simulink model "sim_task_2"  (R2024a)
settings: Solver=FixedStepAuto  StartTime=0.0  StopTime=10.0  FixedStep=1e-3  RelTol=1e-3
settings Model: Creator=alexe  LastModifiedBy=alexe

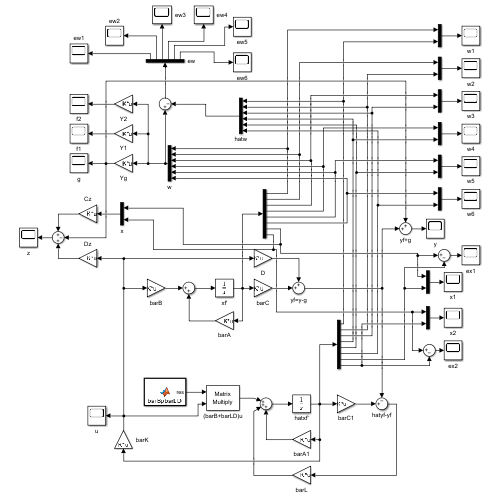
[thumbnail: Simulink's stored preview of the top-level diagram]
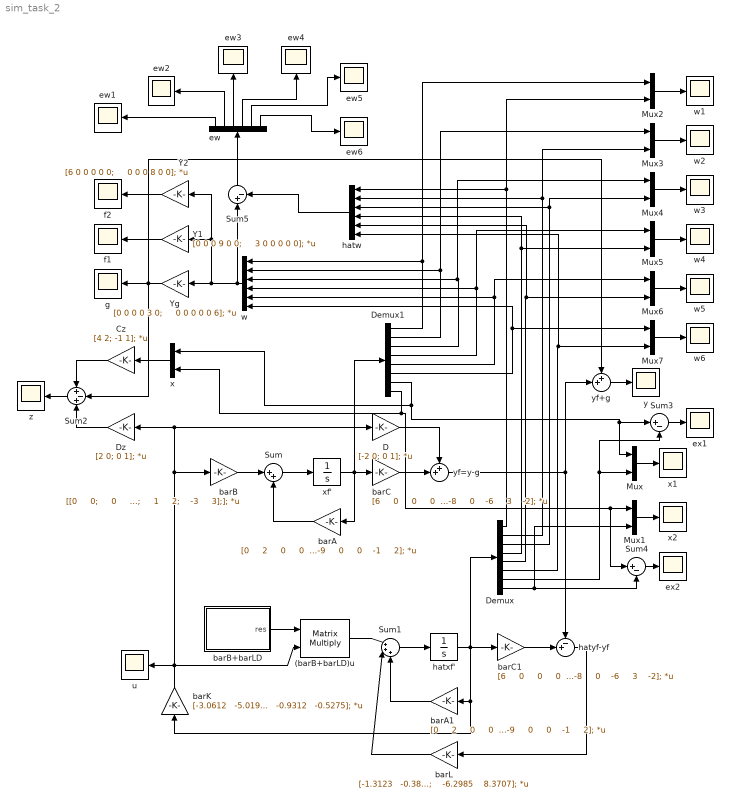
== system sim_task_2 ==
  (barB+barLD)u : Product  Multiplication=Matrix(*)
  Cz : Gain  Gain=[4 2; -1 1];  Multiplication=Matrix(K*u)
  D : Gain  Gain=[-2 0; 0 1];  Multiplication=Matrix(K*u)
  Demux : Demux  Outputs=8
  Demux1 : Demux  Outputs=8
  Dz : Gain  Gain=[2 0; 0 1];  Multiplication=Matrix(K*u)
  Mux{,1..7} (8 alike) : Mux  Inputs=2
  Sum : Sum  Inputs=|++
  Sum1 : Sum  Inputs=|+++
  Sum2 : Sum  Inputs=+-+
  Sum3 : Sum  Inputs=|+-
  Sum4 : Sum  Inputs=|+-
  Sum5 : Sum  Inputs=|+-
  Y1 : Gain  Gain=|  Multiplication=Matrix(K*u)
      | [0 0 0 9 0 0;
      |     3 0 0 0 0 0];
  Y2 : Gain  Gain=|  Multiplication=Matrix(K*u)
      | [6 0 0 0 0 0;
      |     0 0 0 8 0 0];
  Yg : Gain  Gain=|  Multiplication=Matrix(K*u)
      | [0 0 0 0 3 0;
      |     0 0 0 0 0 6];
  barA : Gain  Gain=|  Multiplication=Matrix(K*u)
      | [0     2     0     0     0     0     0     0;
      |     -2     0     0     0     0     0     0     0;
      |      0     0     0     3     0     0     0     0;
      |      0     0    -3     0     0     0     0     0;
      |      0     0     0     0     0     4     0     0;
      |      0     0     0     0    -4     0     0     0;
      |      6     0     0     9     0     0     0     1;
      |      9     0     0    -9     0     0    -1     2];
  barA1 : Gain  Gain=|  Multiplication=Matrix(K*u)
      | [0     2     0     0     0     0     0     0;
      |     -2     0     0     0     0     0     0     0;
      |      0     0     0     3     0     0     0     0;
      |      0     0    -3     0     0     0     0     0;
      |      0     0     0     0     0     4     0     0;
      |      0     0     0     0    -4     0     0     0;
      |      6     0     0     9     0     0     0     1;
      |      9     0     0    -9     0     0    -1     2];
  barB : Gain  Gain=|  Multiplication=Matrix(K*u)
      | [[0     0;
      |     0     0;
      |     0     0;
      |     0     0;
      |     0     0;
      |     0     0;
      |     1     2;
      |    -3     3];];
  barB+barLD : MATLAB Function  TreatAsAtomicUnit=on
  barC : Gain  Gain=|  Multiplication=Matrix(K*u)
      | [6     0     0     0    -3     0     2     1;
      |      0     0     0    -8     0    -6     3    -2];
  barC1 : Gain  Gain=|  Multiplication=Matrix(K*u)
      | [6     0     0     0    -3     0     2     1;
      |      0     0     0    -8     0    -6     3    -2];
  barK : Gain  Gain=|  Multiplication=Matrix(K*u)
      | [-3.0612   -5.0195    7.9863  -12.7069   12.2869   20.2823   -0.8523    0.9009;
      |    -6.4128   -0.9151   -2.9433   -7.3826   17.6422   -0.5952   -0.9312   -0.5275];
  barL : Gain  Gain=|  Multiplication=Matrix(K*u)
      | [-1.3123   -0.3869;
      |    -0.3266   -0.1466;
      |     0.4381   -0.5637;
      |     0.3777   -1.1609;
      |    -0.4550   -0.5493;
      |     1.2212   -0.0019;
      |    -0.3758   -3.2880;
      |    -6.2985    8.3707];
  ew : Demux  Outputs=6
  ew{1..6} (6 alike) : Scope
  ex1 : Scope
  ex2 : Scope
  f1 : Scope
  f2 : Scope
  g : Scope
  hatw : Mux  Inputs=6
  hatxf' : Integrator  InitialCondition=[0;0;0;0;0;0;0;0];
  hatyf-yf : Sum  Inputs=-+|
  u : Scope
  w : Mux  Inputs=6
  w{1..6} (6 alike) : Scope
  x : Mux  Inputs=2
  x1 : Scope
  x2 : Scope
  xf' : Integrator  InitialCondition=[1;0;1;0;1;0;1;1];
  y : Scope
  yf+g : Sum  Inputs=++|
  yf=y-g : Sum  Inputs=++|
  z : Scope
  wires:
  barB/1 -> Sum/1
  Sum/1 -> xf'/1
  barA/1 -> Sum/2
  xf'/1 -> Demux1/1, barC/1, barA/1
  barC/1 -> yf=y-g/2
  D/1 -> yf=y-g/1
  barK/1 -> (barB+barLD)u/2, u/1, barB/1, Dz/1, D/1
  hatxf'/1 -> Demux/1, barK/1, barA1/1, barC1/1
  Sum1/1 -> hatxf'/1
  barA1/1 -> Sum1/3
  (barB+barLD)u/1 -> Sum1/1
  barB+barLD/1(res) -> (barB+barLD)u/1
  hatyf-yf/1 -> barL/1
  barL/1 -> Sum1/2
  barC1/1 -> hatyf-yf/2
  x/1 -> Cz/1
  Demux1/7 -> Sum3/1, Mux/1, x/1
  Demux1/8 -> Sum4/1, Mux1/1, x/2
  Dz/1 -> Sum2/3
  Cz/1 -> Sum2/1
  Sum2/1 -> z/1
  Demux1/1 -> Mux2/1, w/1
  Demux1/2 -> Mux3/1, w/2
  Demux1/3 -> Mux4/1, w/3
  Demux1/4 -> w/4, Mux5/1
  Demux1/5 -> w/5, Mux6/1
  Demux1/6 -> Mux7/1, w/6
  w/1 -> Sum5/1, Y2/1, Y1/1, Yg/1
  Yg/1 -> yf+g/1, g/1, Sum2/2
  Y1/1 -> f1/1
  Y2/1 -> f2/1
  yf=y-g/1 -> hatyf-yf/1, yf+g/2
  yf+g/1 -> y/1
  Demux/7 -> Mux/2, Sum3/2
  Mux/1 -> x1/1
  Demux/8 -> Sum4/2, Mux1/2
  Mux1/1 -> x2/1
  Sum3/1 -> ex1/1
  Sum4/1 -> ex2/1
  Demux/1 -> Mux2/2, hatw/1
  Mux2/1 -> w1/1
  Demux/2 -> Mux3/2, hatw/2
  Mux3/1 -> w2/1
  Mux4/1 -> w3/1
  Demux/3 -> hatw/3, Mux4/2
  Mux5/1 -> w4/1
  Demux/4 -> hatw/4, Mux5/2
  Mux6/1 -> w5/1
  Demux/5 -> hatw/5, Mux6/2
  Mux7/1 -> w6/1
  Demux/6 -> hatw/6, Mux7/2
  hatw/1 -> Sum5/2
  Sum5/1 -> ew/1
  ew/1 -> ew1/1
  ew/2 -> ew2/1
  ew/3 -> ew3/1
  ew/4 -> ew4/1
  ew/5 -> ew5/1
  ew/6 -> ew6/1

== matlab function sim_task_2/barB+barLD ==
  data: res output
function res = barBpbarLD()

bB=[0     0;
    0     0;
    0     0;
    0     0;
    0     0;
    0     0;
    1     2;
   -3     3];
bL=[-1.3123   -0.3869;
   -0.3266   -0.1466;
    0.4381   -0.5637;
    0.3777   -1.1609;
   -0.4550   -0.5493;
    1.2212   -0.0019;
   -0.3758   -3.2880;
   -6.2985    8.3707];
D=[-2 0; 0 1];

res = [bB+bL*D];

end
